simulink model "inducmotor"  (R2025a)
settings: Solver=VariableStepAuto  StartTime=0.0  StopTime=10.0  RelTol=1e-3
libraries: simulink x4, spsAsynchronousMachinepuUnitsLib x1, spsDCVoltageSourceLib x1, eePwmGeneratorTwoLevel x1, spsThreePhaseVIMeasurementLib x1, spsUniversalBridgeLib x1, spsVoltageMeasurementLib x1, sps_lib x1
settings Model: Creator=anirudh  LastModifiedBy=anirudh
settings DataIOCC: ReturnWorkspaceOutputs=off

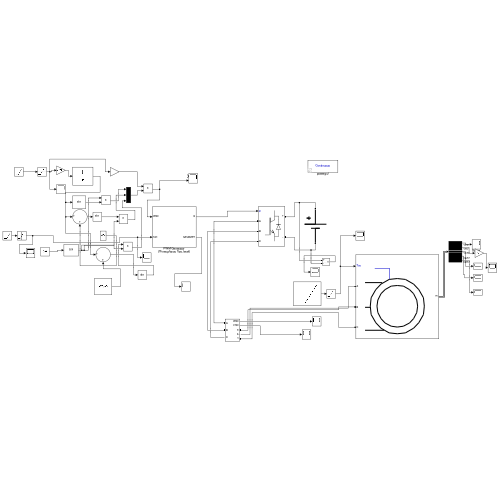
[thumbnail: Simulink's stored preview of the top-level diagram]
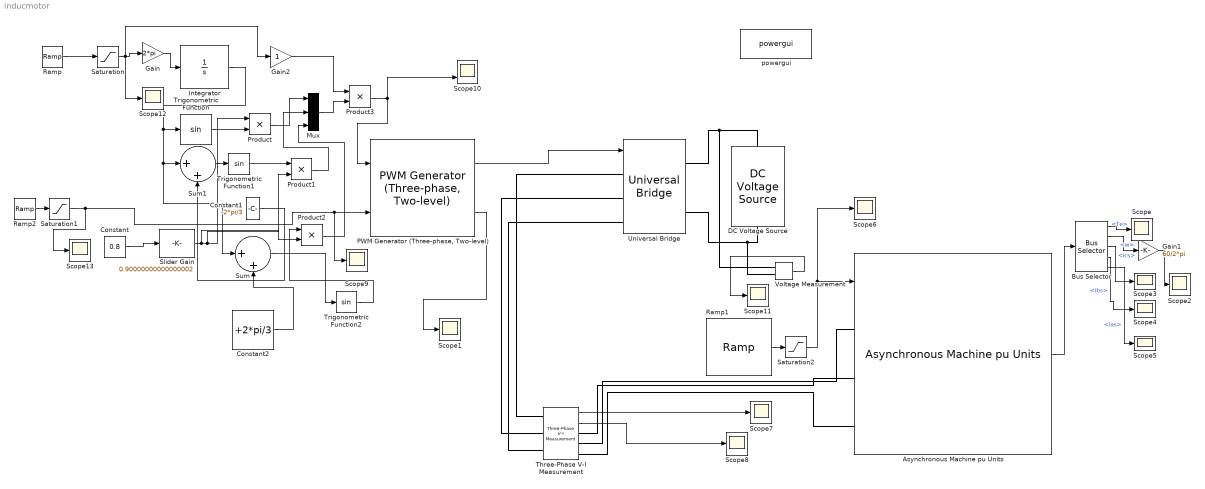
== system inducmotor ==
  Asynchronous Machine pu Units : spsAsynchronousMachinepuUnitsLib/Asynchronous Machine pu Units  RotorType=Squirrel-cage  PresetModel=No  MechanicalLoad=Torque Tm  ShowDetailedParameters=on  ReferenceFrame=Rotor  Units=pu  MeasurementBus=on  NominalParameters=[3730 460 60]  VoltageRatio=1  Stator=[0.01965 0.0397]  Rotor=[0.01909 0.0397]  Cage1=[0.01909 0.0397]  Cage2=[0.01909 0.0397]  Lm=1.354  Mechanical=[0.09526 0.05479 2]  PolePairs=2  InitialConditions="[ 1,0   0,0,0   0,0,0 ]"  SimulateSaturation=off  Saturation="[0.212,0.4201,0.8125,1.0979,1.4799,2.2457,3.2586,4.5763,6.4763 ;   0.5,0.7,0.9,1,1.1,1.2 ,1.3,1.4,1.5]"  LoadFlowParameters=0  TsPowergui=0  TsBlock=-1  IterativeModel=Trapezoidal non iterative  IterativeDiscreteModel=Trapezoidal non iterative  Pmec=0
      settings: LibrarySourceBlock=|
      | sps_lib/Electrical Machines/Asynchronous Machine
      | pu Units
  Bus Selector : BusSelector  OutputSignals=Te,w,ics,ibs,ias
  Constant : Constant  Value=0.8
  Constant1 : Constant  Value=-2*pi/3
  Constant2 : Constant  Value=+2*pi/3
  DC Voltage Source : spsDCVoltageSourceLib/DC Voltage Source  Amplitude=600  Measurements=None
  Gain : Gain  Gain=2*pi
  Gain1 : Gain  Gain=60/2*pi
  Gain2 : Gain
  Integrator : Integrator
  Mux : Mux  Inputs=3
  "PWM Generator (Three-phase, Two-level)" : eePwmGeneratorTwoLevel/PWM Generator (Three-phase, Two-level)  PWMMode=Continuous PWM (CPWM)  CPWMMode=SPWM: sinusoidal PWM  DPWMMode=60 DPWM: 60 degree discontinuous PWM  fsw=1e3  Ts=5e-5
      settings: LibrarySourceBlock=|
      | ee_sl_lib/Pulse Width
      | Modulation/PWM Generator
      | (Three-phase, Two-level)
  Product{,1..3} (4 alike) : Product
  Ramp : simulink/Sources/Ramp  slope=12.5  start=0  InitialOutput=0
  Ramp1 : simulink/Sources/Ramp  slope=0.5  start=3  InitialOutput=0
  Ramp2 : simulink/Sources/Ramp  slope=200  start=0  InitialOutput=0
  Saturation : Saturate  UpperLimit=50  LowerLimit=0
  Saturation1 : Saturate  UpperLimit=600  LowerLimit=0
  Saturation2 : Saturate  UpperLimit=0.8  LowerLimit=0
  Scope{,1..9,11..13} (13 alike) : Scope
      Scope settings: ActiveDisplayYMinimum=-2.0966468722959131  ActiveDisplayYMaximum=2.55807645218612  DataLoggingVariableName=torquescope
      Scope1 settings: ActiveDisplayYMinimum=-0.15000000000000027  ActiveDisplayYMaximum=0.15000000000000038
      Scope11 settings: ActiveDisplayYMinimum=-1  ActiveDisplayYMaximum=1  DataLoggingVariableName=ScopeData11
      Scope12 settings: ActiveDisplayYMinimum=-303.0159453245202  ActiveDisplayYMaximum=61.38422938299469  DataLoggingVariableName=ScopeData12
      Scope13 settings: ActiveDisplayYMinimum=-1  ActiveDisplayYMaximum=1  DataLoggingVariableName=ScopeData13
      Scope2 settings: ActiveDisplayYMinimum=-1  ActiveDisplayYMaximum=1  DataLoggingVariableName=wscope
      Scope3 settings: ActiveDisplayYMinimum=-1  ActiveDisplayYMaximum=1  DataLoggingVariableName=ScopeData3
      Scope4 settings: ActiveDisplayYMinimum=-4.5303480378514083  ActiveDisplayYMaximum=3.7295122250457919  DataLoggingVariableName=ScopeData4
      Scope5 settings: ActiveDisplayYMinimum=-1  ActiveDisplayYMaximum=1  DataLoggingVariableName=ScopeData5
      Scope6 settings: ActiveDisplayYMinimum=-1  ActiveDisplayYMaximum=1  DataLoggingVariableName=ScopeData6
      Scope7 settings: ActiveDisplayYMinimum=-737.53660206607333  ActiveDisplayYMaximum=734.83985958752589  DataLoggingVariableName=ScopeData7
      Scope8 settings: ActiveDisplayYMinimum=-137.93008907930533  ActiveDisplayYMaximum=161.35000171429678  DataLoggingVariableName=iabcscope
      Scope9 settings: ActiveDisplayYMinimum=-1  ActiveDisplayYMaximum=1  DataLoggingVariableName=vdcscope
  Scope10 : Scope  NumInputPorts=2
      settings: ActiveDisplayYMinimum=-1  ActiveDisplayYMaximum=1  DataLoggingVariableName=vabcscope
  Slider Gain : simulink/Math Operations/Slider Gain  gain=0.90000000000000002  low=0.2  high=0.9
  Sum : Sum  Inputs=|++
  Sum1 : Sum  Inputs=|++
  Three-Phase V-I Measurement : spsThreePhaseVIMeasurementLib/Three-Phase V-I Measurement  VoltageMeasurement=phase-to-phase  SetLabelV=off  LabelV=Vabc  Vpu=off  VpuLL=off  CurrentMeasurement=yes  SetLabelI=off  LabelI=Iabc  Ipu=off  Pbase=100e6  Vbase=500e3  OutputType=Complex  PhasorSimulation=off  PSBequivalent=0
  Trigonometric Function : Trigonometry
  Trigonometric Function1 : Trigonometry
  Trigonometric Function2 : Trigonometry
  Universal Bridge : spsUniversalBridgeLib/Universal Bridge  Arms=3  SnubberResistance=1e5  SnubberCapacitance=inf  Device=IGBT / Diodes  Ron=1e-3  Lon=0  ForwardVoltages="[  0  0  ]"  ForwardVoltage=0  GTOparameters=[ 10e-6 , 20e-6 ]  IGBTparameters=[ 1e-6 , 2e-6 ]  Measurements=None  Measurements_2=None  converterType=Rectifier
  Voltage Measurement : spsVoltageMeasurementLib/Voltage Measurement  PhasorSimulation=off  OutputType=Complex  PSBequivalent=0
  powergui : sps_lib/powergui  Priority=1  SimulationMode=Continuous  SampleTime=50e-6  frequency=60  Iterations=50  frequencyindice=60  Pbase=100e6  ErrMax=1e-4  UnitsV=kV  UnitsW=MW  buscounter=0  FunctionMessages=off  echomessages=off  EnableUseOfTLC=off  CurrentSourceSwitches=off  DisableSnubberDevices=off  DisableRonSwitches=off  DisableVfSwitches=off  DisplayEquations=off  AutomaticDiscreteSolvers=off  SolverType=Tustin/Backward Euler (TBE)  Interpol=off  ExternalGateDelay=off  methode=off  Ts=100  x0status=blocks  SPID=on  SwTol=0  HookPort=off  NonlinearTolerance=1e-4  nMaxIteration=100  ContinueOnMaxIteration=off  RestoreLinks=warning  ResistiveCurrentMeasurement=off  Frange=[0:2:500]  Ylog=off  Xlog=on  ShowGrid=off  save=off  variable=ZData  structure=0  ZoomFFT=off  StartTime=0.0  cycles=1  DisplayStyle=1  fundamental=60  FreqAxis=off  MaxFrequency=1000  frequencyindicesteady=1  RmsSteady=1  display=off
  wires:
  "PWM Generator (Three-phase, Two-level)"/1 -> Universal Bridge/1
  Gain/1 -> Integrator/1
  Constant1/1 -> Sum1/2
  Integrator/1 -> Sum/1, Sum1/1, Trigonometric Function/1
  Constant2/1 -> Sum/2
  Ramp2/1 -> Saturation1/1
  Slider Gain/1 -> Product2/2, Product1/2, Product/1
  Trigonometric Function/1 -> Product/2
  Product/1 -> Mux/1
  Product1/1 -> Mux/2
  Product2/1 -> Mux/3
  "PWM Generator (Three-phase, Two-level)"/2 -> Scope1/1
  Ramp1/1 -> Saturation2/1
  Asynchronous Machine pu Units/1 -> Bus Selector/1
  Bus Selector/1 -> Scope/1  "<Te>"
  Bus Selector/3 -> Scope3/1  "<ics>"
  Bus Selector/4 -> Scope4/1  "<ibs>"
  Bus Selector/5 -> Scope5/1  "<ias>"
  Three-Phase V-I Measurement/1 -> Scope7/1
  Three-Phase V-I Measurement/2 -> Scope8/1
  Voltage Measurement/1 -> Scope11/1
  Bus Selector/2 -> Gain1/1  "<w>"
  Gain1/1 -> Scope2/1
  Constant/1 -> Slider Gain/1
  Mux/1 -> Product3/2
  Gain2/1 -> Product3/1
  Product3/1 -> "PWM Generator (Three-phase, Two-level)"/1, Scope10/2
  Ramp/1 -> Saturation/1
  Saturation/1 -> Gain2/1, Scope12/1, Gain/1
  Sum1/1 -> Trigonometric Function1/1
  Trigonometric Function1/1 -> Product1/1
  Sum/1 -> Trigonometric Function2/1
  Trigonometric Function2/1 -> Product2/1
  Saturation1/1 -> Scope13/1, "PWM Generator (Three-phase, Two-level)"/2, Scope9/1
  Saturation2/1 -> Scope6/1, Asynchronous Machine pu Units/1
  connections:
  Universal Bridge/RConn1 -- DC Voltage Source/RConn1 -- Voltage Measurement/LConn1
  Universal Bridge/RConn2 -- Voltage Measurement/LConn2 -- DC Voltage Source/LConn1
  Three-Phase V-I Measurement/RConn3 -- Asynchronous Machine pu Units/LConn3
  Universal Bridge/LConn1 -- Three-Phase V-I Measurement/LConn1
  Universal Bridge/LConn2 -- Three-Phase V-I Measurement/LConn2
  Universal Bridge/LConn3 -- Three-Phase V-I Measurement/LConn3
  Three-Phase V-I Measurement/RConn1 -- Asynchronous Machine pu Units/LConn2
  Three-Phase V-I Measurement/RConn2 -- Asynchronous Machine pu Units/LConn1
